simulink model "TrofazniTiristorskiIspravljac2"  (R2014b)
settings: Solver=ode5  StartTime=0.0  StopTime=0.1  FixedStep=10e-6  RelTol=1e-3
values from neighbouring files (symbols this model uses):
  alfa = 60    [ParametriSimulacije.m]
  f = 50    [ParametriSimulacije.m]
  L = 20e-3    (= 0.02)    [ParametriSimulacije.m]
  R = 10    [ParametriSimulacije.m]
  Vmax = 220*sqrt(2)    [ParametriSimulacije.m]
libraries: powerlib x13
settings Model: Creator=Zorana  LastModifiedBy=Zorana

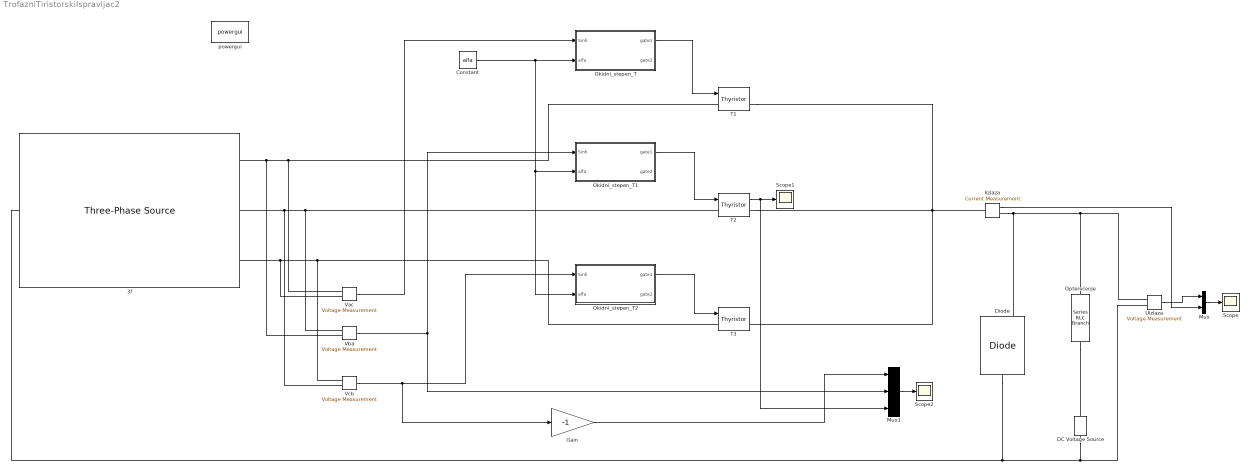
== system TrofazniTiristorskiIspravljac2 ==
  3f : powerlib/Electrical Sources/Three-Phase Source  Voltage=380  PhaseAngle=0  Frequency=f  InternalConnection=Yn  SpecifyImpedance=off  Resistance=1e-6  Inductance=0  ShortCircuitLevel=100e6  BaseVoltage=25e3  XRratio=7  BusType=swing  Pref=0  Qref=0  Qmin=-inf  Qmax=inf
  Constant : Constant  Value=alfa
  DC Voltage Source : powerlib/Electrical Sources/DC Voltage Source  Amplitude=50  Measurements=None
  Diode : powerlib/Power Electronics/Diode  Ron=1e-6  Lon=0  Vf=0  IC=0  UseSnubber=off  Rs=500  Cs=250e-9  Measurements=on
  Gain : Gain  Gain=-1
  Iizlaza : powerlib/Measurements/Current Measurement  PhasorSimulation=off  OutputType=Complex  PSBequivalent=0
  Mux : Mux  Inputs=2
  Mux1 : Mux  Inputs=3
  Okidni_stepen_T : Subsystem
  Okidni_stepen_T1 : Subsystem
  Okidni_stepen_T2 : Subsystem
  Opterećenje : powerlib/Elements/Series RLC Branch  LConnTagsString=__new0  RConnTagsString=__new0  BranchType=RL  Resistance=R  Inductance=L  SetiL0=off  InitialCurrent=0  Capacitance=1e-6  Setx0=off  InitialVoltage=0  Measurements=None
  Scope : Scope
  Scope1 : Scope
  Scope2 : Scope
      settings: SaveName=ScopeData2
  T1 : powerlib/Power Electronics/Thyristor  Ron=1e-6  Lon=0  Vf=0  IC=0  Rs=500  Cs=250e-9  Measurements=on
  T2 : powerlib/Power Electronics/Thyristor  Ron=1e-6  Lon=0  Vf=0  IC=0  Rs=500  Cs=250e-9  Measurements=on
  T3 : powerlib/Power Electronics/Thyristor  Ron=1e-6  Lon=0  Vf=0  IC=0  Rs=500  Cs=250e-9  Measurements=on
  Uizlaza : powerlib/Measurements/Voltage Measurement  PhasorSimulation=off  OutputType=Complex  PSBequivalent=0
  Vac : powerlib/Measurements/Voltage Measurement  PhasorSimulation=off  OutputType=Complex  PSBequivalent=0
  Vba : powerlib/Measurements/Voltage Measurement  PhasorSimulation=off  OutputType=Complex  PSBequivalent=0
  Vcb : powerlib/Measurements/Voltage Measurement  PhasorSimulation=off  OutputType=Complex  PSBequivalent=0
  powergui : powerlib/powergui  Priority=1  SimulationMode=Continuous  SolverType=Tustin/Backward Euler (TBE)  SampleTime=50e-6  frequency=60  SPID=off  DisableSnubberDevices=off  DisableRonSwitches=off  DisableVfSwitches=off  SwTol=0  DisplayEquations=off  Interpol=off  methode=off  Ts=100  frequencyindice=50  Pbase=100e6  ErrMax=1e-4  Iterations=50  UnitsV=kV  UnitsW=MW  FunctionMessages=off  echomessages=off  HookPort=off  EnableUseOfTLC=off  x0status=blocks  RestoreLinks=warning  ResistiveCurrentMeasurement=off  Frange=[0:2:500]  Ylog=off  Xlog=on  ShowGrid=off  save=off  variable=ZData  structure=0  ZoomFFT=off  StartTime=0.0  cycles=1  DisplayStyle=1  fundamental=60  FreqAxis=off  MaxFrequency=1000  frequencyindicesteady=1  RmsSteady=1  display=off
  wires:
  Constant/1 -> Okidni_stepen_T2/2(alfa), Okidni_stepen_T1/2(alfa), Okidni_stepen_T/2(alfa)
  Okidni_stepen_T/1(gate1) -> T1/1
  Okidni_stepen_T1/1(gate1) -> T2/1
  Okidni_stepen_T2/1(gate1) -> T3/1
  Vac/1 -> Okidni_stepen_T/1(Sinh)
  Vba/1 -> Okidni_stepen_T1/1(Sinh), Mux1/2
  Vcb/1 -> Gain/1, Okidni_stepen_T2/1(Sinh)
  Uizlaza/1 -> Mux/1
  Mux/1 -> Scope/1
  Iizlaza/1 -> Mux/2
  T2/1 -> Mux1/3, Scope1/1
  Mux1/1 -> Scope2/1
  Gain/1 -> Mux1/1
  connections:
  T1/LConn1 -- Vac/LConn1 -- Vba/LConn2 -- 3f/RConn1
  T2/LConn1 -- Vba/LConn1 -- 3f/RConn2 -- Vcb/LConn2
  T3/LConn1 -- Vcb/LConn1 -- Vac/LConn2 -- 3f/RConn3
  T1/RConn1 -- Iizlaza/LConn1 -- T2/RConn1 -- T3/RConn1
  Uizlaza/LConn2 -- DC Voltage Source/LConn1 -- Diode/LConn1 -- 3f/LConn1
  Iizlaza/RConn1 -- Uizlaza/LConn1 -- Opterećenje/LConn1 -- Diode/RConn1
  Opterećenje/RConn1 -- DC Voltage Source/RConn1

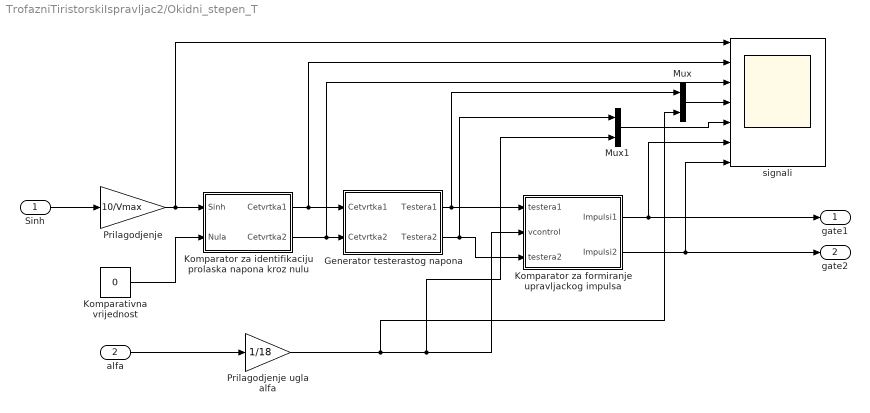
== system TrofazniTiristorskiIspravljac2/Okidni_stepen_T ==
  Sinh : Inport
  alfa : Inport  Port=2
  Generator testerastog napona : Subsystem
  Komparativna vrijednost : Constant  Value=0
  Komparator za formiranje upravljackog impulsa : Subsystem
  Komparator za identifikaciju prolaska napona kroz nulu : Subsystem
  Mux : Mux  Inputs=2
  Mux1 : Mux  Inputs=2
  Prilagodjenje : Gain  Gain=10/Vmax
  Prilagodjenje ugla alfa : Gain  Gain=1/18
  signali : Scope  NumInputPorts=7
      settings: YMin=-10~0~0~0~-5~0~0  YMax=10~11~11~11~5~11~11  SaveName=ScopeData3
  gate1 : Outport
  gate2 : Outport  Port=2
  wires:
  Komparator za formiranje upravljackog impulsa/1(Impulsi1) -> signali/6, gate1/1
  Komparator za identifikaciju prolaska napona kroz nulu/1(Cetvrtka1) -> signali/2, Generator testerastog napona/1(Cetvrtka1)
  Sinh/1 -> Prilagodjenje/1
  Prilagodjenje ugla alfa/1 -> Mux/2, Mux1/2, Komparator za formiranje upravljackog impulsa/2(vcontrol)
  Prilagodjenje/1 -> signali/1, Komparator za identifikaciju prolaska napona kroz nulu/1(Sinh)
  Generator testerastog napona/1(Testera1) -> Mux/1, Komparator za formiranje upravljackog impulsa/1(testera1)
  alfa/1 -> Prilagodjenje ugla alfa/1
  Komparativna vrijednost/1 -> Komparator za identifikaciju prolaska napona kroz nulu/2(Nula)
  Komparator za identifikaciju prolaska napona kroz nulu/2(Cetvrtka2) -> signali/3, Generator testerastog napona/2(Cetvrtka2)
  Generator testerastog napona/2(Testera2) -> Mux1/1, Komparator za formiranje upravljackog impulsa/3(testera2)
  Komparator za formiranje upravljackog impulsa/2(Impulsi2) -> signali/7, gate2/1
  Mux/1 -> signali/4
  Mux1/1 -> signali/5

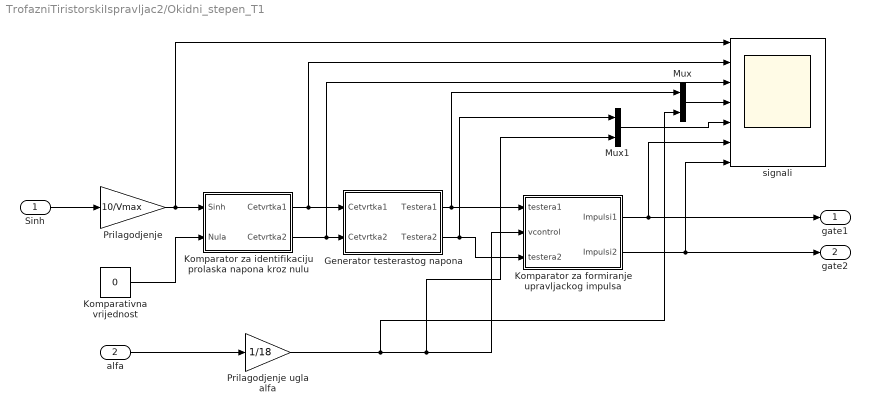
== system TrofazniTiristorskiIspravljac2/Okidni_stepen_T1 ==
  Sinh : Inport
  alfa : Inport  Port=2
  Generator testerastog napona : Subsystem
  Komparativna vrijednost : Constant  Value=0
  Komparator za formiranje upravljackog impulsa : Subsystem
  Komparator za identifikaciju prolaska napona kroz nulu : Subsystem
  Mux : Mux  Inputs=2
  Mux1 : Mux  Inputs=2
  Prilagodjenje : Gain  Gain=10/Vmax
  Prilagodjenje ugla alfa : Gain  Gain=1/18
  signali : Scope  NumInputPorts=7
      settings: YMin=-10~0~0~0~-5~0~0  YMax=10~11~11~11~5~11~11  SaveName=ScopeData3
  gate1 : Outport
  gate2 : Outport  Port=2
  wires:
  Mux1/1 -> signali/5
  Mux/1 -> signali/4
  Komparator za formiranje upravljackog impulsa/2(Impulsi2) -> gate2/1, signali/7
  Generator testerastog napona/2(Testera2) -> Komparator za formiranje upravljackog impulsa/3(testera2), Mux1/1
  Komparator za identifikaciju prolaska napona kroz nulu/2(Cetvrtka2) -> Generator testerastog napona/2(Cetvrtka2), signali/3
  Komparativna vrijednost/1 -> Komparator za identifikaciju prolaska napona kroz nulu/2(Nula)
  alfa/1 -> Prilagodjenje ugla alfa/1
  Generator testerastog napona/1(Testera1) -> Komparator za formiranje upravljackog impulsa/1(testera1), Mux/1
  Prilagodjenje/1 -> Komparator za identifikaciju prolaska napona kroz nulu/1(Sinh), signali/1
  Prilagodjenje ugla alfa/1 -> Komparator za formiranje upravljackog impulsa/2(vcontrol), Mux1/2, Mux/2
  Sinh/1 -> Prilagodjenje/1
  Komparator za identifikaciju prolaska napona kroz nulu/1(Cetvrtka1) -> Generator testerastog napona/1(Cetvrtka1), signali/2
  Komparator za formiranje upravljackog impulsa/1(Impulsi1) -> gate1/1, signali/6

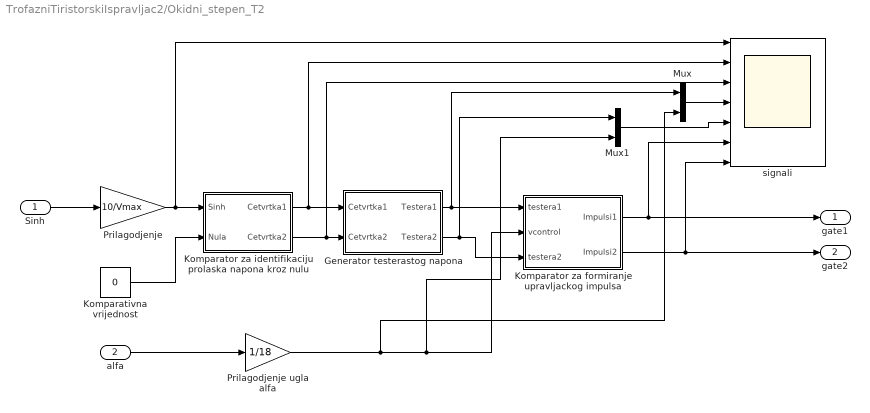
== system TrofazniTiristorskiIspravljac2/Okidni_stepen_T2 ==
  Sinh : Inport
  alfa : Inport  Port=2
  Generator testerastog napona : Subsystem
  Komparativna vrijednost : Constant  Value=0
  Komparator za formiranje upravljackog impulsa : Subsystem
  Komparator za identifikaciju prolaska napona kroz nulu : Subsystem
  Mux : Mux  Inputs=2
  Mux1 : Mux  Inputs=2
  Prilagodjenje : Gain  Gain=10/Vmax
  Prilagodjenje ugla alfa : Gain  Gain=1/18
  signali : Scope  NumInputPorts=7
      settings: YMin=-10~0~0~0~-5~0~0  YMax=10~11~11~11~5~11~11  SaveName=ScopeData3
  gate1 : Outport
  gate2 : Outport  Port=2
  wires:
  Komparator za formiranje upravljackog impulsa/1(Impulsi1) -> signali/6, gate1/1
  Komparator za identifikaciju prolaska napona kroz nulu/1(Cetvrtka1) -> signali/2, Generator testerastog napona/1(Cetvrtka1)
  Sinh/1 -> Prilagodjenje/1
  Prilagodjenje ugla alfa/1 -> Mux/2, Mux1/2, Komparator za formiranje upravljackog impulsa/2(vcontrol)
  Prilagodjenje/1 -> signali/1, Komparator za identifikaciju prolaska napona kroz nulu/1(Sinh)
  Generator testerastog napona/1(Testera1) -> Mux/1, Komparator za formiranje upravljackog impulsa/1(testera1)
  alfa/1 -> Prilagodjenje ugla alfa/1
  Komparativna vrijednost/1 -> Komparator za identifikaciju prolaska napona kroz nulu/2(Nula)
  Komparator za identifikaciju prolaska napona kroz nulu/2(Cetvrtka2) -> signali/3, Generator testerastog napona/2(Cetvrtka2)
  Generator testerastog napona/2(Testera2) -> Mux1/1, Komparator za formiranje upravljackog impulsa/3(testera2)
  Komparator za formiranje upravljackog impulsa/2(Impulsi2) -> signali/7, gate2/1
  Mux/1 -> signali/4
  Mux1/1 -> signali/5

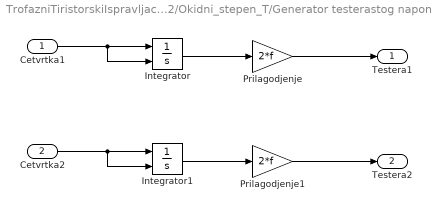
== system TrofazniTiristorskiIspravljac2/Okidni_stepen_T/Generator testerastog napona ==
  Cetvrtka1 : Inport
  Cetvrtka2 : Inport  Port=2
  Integrator : Integrator  ExternalReset=either
  Integrator1 : Integrator  ExternalReset=either
  Prilagodjenje : Gain  Gain=2*f
  Prilagodjenje1 : Gain  Gain=2*f
  Testera1 : Outport
  Testera2 : Outport  Port=2
  wires:
  Integrator/1 -> Prilagodjenje/1
  Cetvrtka1/1 -> Integrator/1, Integrator/2
  Prilagodjenje/1 -> Testera1/1
  Integrator1/1 -> Prilagodjenje1/1
  Cetvrtka2/1 -> Integrator1/2, Integrator1/1
  Prilagodjenje1/1 -> Testera2/1

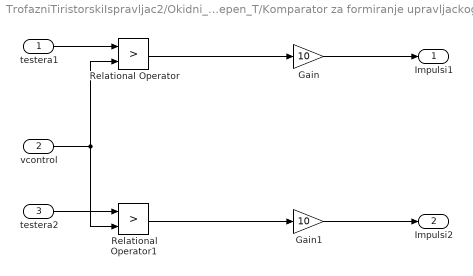
== system TrofazniTiristorskiIspravljac2/Okidni_stepen_T/Komparator za formiranje upravljackog impulsa ==
  testera1 : Inport
  vcontrol : Inport  Port=2
  testera2 : Inport  Port=3
  Gain : Gain  Gain=10
  Gain1 : Gain  Gain=10
  Relational Operator : RelationalOperator  Operator=>  OutDataTypeStr=fixdt(1,16)  InputSameDT=on
  Relational Operator1 : RelationalOperator  Operator=>  OutDataTypeStr=fixdt(1,16)  InputSameDT=on
  Impulsi1 : Outport
  Impulsi2 : Outport  Port=2
  wires:
  vcontrol/1 -> Relational Operator/2, Relational Operator1/2
  testera1/1 -> Relational Operator/1
  Gain/1 -> Impulsi1/1
  testera2/1 -> Relational Operator1/1
  Gain1/1 -> Impulsi2/1
  Relational Operator/1 -> Gain/1
  Relational Operator1/1 -> Gain1/1

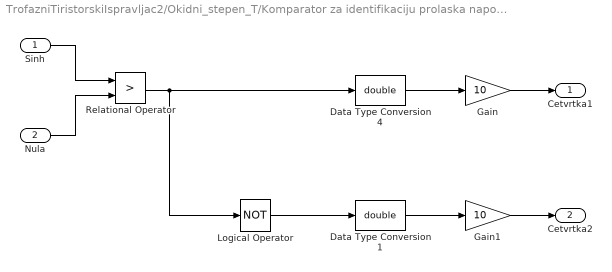
== system TrofazniTiristorskiIspravljac2/Okidni_stepen_T/Komparator za identifikaciju prolaska napona kroz nulu ==
  Sinh : Inport
  Nula : Inport  Port=2
  Data Type Conversion1 : DataTypeConversion  OutDataTypeStr=double  SaturateOnIntegerOverflow=on  RndMeth=Zero
  Data Type Conversion4 : DataTypeConversion  OutDataTypeStr=double  SaturateOnIntegerOverflow=on  RndMeth=Zero
  Gain : Gain  Gain=10
  Gain1 : Gain  Gain=10
  Logical Operator : Logic  Operator=NOT  IconShape=distinctive  AllPortsSameDT=off  OutDataTypeStr=boolean
  Relational Operator : RelationalOperator  Operator=>  OutDataTypeStr=fixdt(1,16)  InputSameDT=on
  Cetvrtka1 : Outport
  Cetvrtka2 : Outport  Port=2
  wires:
  Gain/1 -> Cetvrtka1/1
  Sinh/1 -> Relational Operator/1
  Nula/1 -> Relational Operator/2
  Relational Operator/1 -> Logical Operator/1, Data Type Conversion4/1
  Data Type Conversion4/1 -> Gain/1
  Gain1/1 -> Cetvrtka2/1
  Data Type Conversion1/1 -> Gain1/1
  Logical Operator/1 -> Data Type Conversion1/1

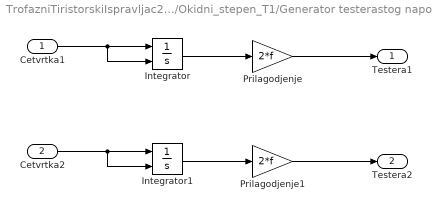
== system TrofazniTiristorskiIspravljac2/Okidni_stepen_T1/Generator testerastog napona ==
  Cetvrtka1 : Inport
  Cetvrtka2 : Inport  Port=2
  Integrator : Integrator  ExternalReset=either
  Integrator1 : Integrator  ExternalReset=either
  Prilagodjenje : Gain  Gain=2*f
  Prilagodjenje1 : Gain  Gain=2*f
  Testera1 : Outport
  Testera2 : Outport  Port=2
  wires:
  Prilagodjenje1/1 -> Testera2/1
  Cetvrtka2/1 -> Integrator1/1, Integrator1/2
  Integrator1/1 -> Prilagodjenje1/1
  Prilagodjenje/1 -> Testera1/1
  Cetvrtka1/1 -> Integrator/2, Integrator/1
  Integrator/1 -> Prilagodjenje/1

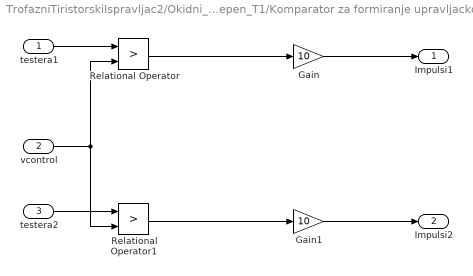
== system TrofazniTiristorskiIspravljac2/Okidni_stepen_T1/Komparator za formiranje upravljackog impulsa ==
  testera1 : Inport
  vcontrol : Inport  Port=2
  testera2 : Inport  Port=3
  Gain : Gain  Gain=10
  Gain1 : Gain  Gain=10
  Relational Operator : RelationalOperator  Operator=>  OutDataTypeStr=fixdt(1,16)  InputSameDT=on
  Relational Operator1 : RelationalOperator  Operator=>  OutDataTypeStr=fixdt(1,16)  InputSameDT=on
  Impulsi1 : Outport
  Impulsi2 : Outport  Port=2
  wires:
  Relational Operator1/1 -> Gain1/1
  Relational Operator/1 -> Gain/1
  Gain1/1 -> Impulsi2/1
  testera2/1 -> Relational Operator1/1
  Gain/1 -> Impulsi1/1
  testera1/1 -> Relational Operator/1
  vcontrol/1 -> Relational Operator1/2, Relational Operator/2

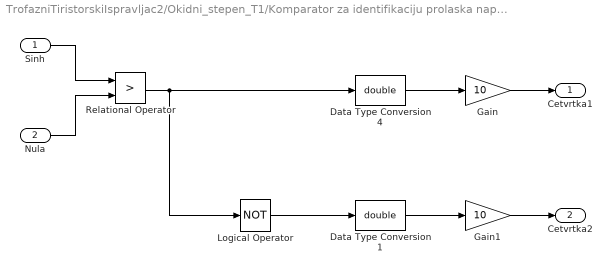
== system TrofazniTiristorskiIspravljac2/Okidni_stepen_T1/Komparator za identifikaciju prolaska napona kroz nulu ==
  Sinh : Inport
  Nula : Inport  Port=2
  Data Type Conversion1 : DataTypeConversion  OutDataTypeStr=double  SaturateOnIntegerOverflow=on  RndMeth=Zero
  Data Type Conversion4 : DataTypeConversion  OutDataTypeStr=double  SaturateOnIntegerOverflow=on  RndMeth=Zero
  Gain : Gain  Gain=10
  Gain1 : Gain  Gain=10
  Logical Operator : Logic  Operator=NOT  IconShape=distinctive  AllPortsSameDT=off  OutDataTypeStr=boolean
  Relational Operator : RelationalOperator  Operator=>  OutDataTypeStr=fixdt(1,16)  InputSameDT=on
  Cetvrtka1 : Outport
  Cetvrtka2 : Outport  Port=2
  wires:
  Logical Operator/1 -> Data Type Conversion1/1
  Data Type Conversion1/1 -> Gain1/1
  Gain1/1 -> Cetvrtka2/1
  Data Type Conversion4/1 -> Gain/1
  Relational Operator/1 -> Data Type Conversion4/1, Logical Operator/1
  Nula/1 -> Relational Operator/2
  Sinh/1 -> Relational Operator/1
  Gain/1 -> Cetvrtka1/1

== system TrofazniTiristorskiIspravljac2/Okidni_stepen_T2/Generator testerastog napona ==
  Cetvrtka1 : Inport
  Cetvrtka2 : Inport  Port=2
  Integrator : Integrator  ExternalReset=either
  Integrator1 : Integrator  ExternalReset=either
  Prilagodjenje : Gain  Gain=2*f
  Prilagodjenje1 : Gain  Gain=2*f
  Testera1 : Outport
  Testera2 : Outport  Port=2
  wires:
  Integrator/1 -> Prilagodjenje/1
  Cetvrtka1/1 -> Integrator/1, Integrator/2
  Prilagodjenje/1 -> Testera1/1
  Integrator1/1 -> Prilagodjenje1/1
  Cetvrtka2/1 -> Integrator1/2, Integrator1/1
  Prilagodjenje1/1 -> Testera2/1

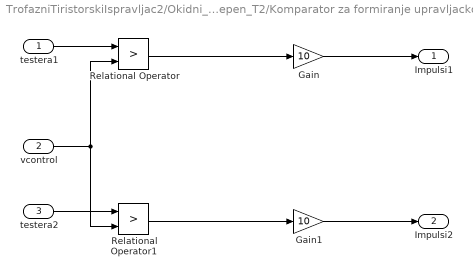
== system TrofazniTiristorskiIspravljac2/Okidni_stepen_T2/Komparator za formiranje upravljackog impulsa ==
  testera1 : Inport
  vcontrol : Inport  Port=2
  testera2 : Inport  Port=3
  Gain : Gain  Gain=10
  Gain1 : Gain  Gain=10
  Relational Operator : RelationalOperator  Operator=>  OutDataTypeStr=fixdt(1,16)  InputSameDT=on
  Relational Operator1 : RelationalOperator  Operator=>  OutDataTypeStr=fixdt(1,16)  InputSameDT=on
  Impulsi1 : Outport
  Impulsi2 : Outport  Port=2
  wires:
  vcontrol/1 -> Relational Operator/2, Relational Operator1/2
  testera1/1 -> Relational Operator/1
  Gain/1 -> Impulsi1/1
  testera2/1 -> Relational Operator1/1
  Gain1/1 -> Impulsi2/1
  Relational Operator/1 -> Gain/1
  Relational Operator1/1 -> Gain1/1

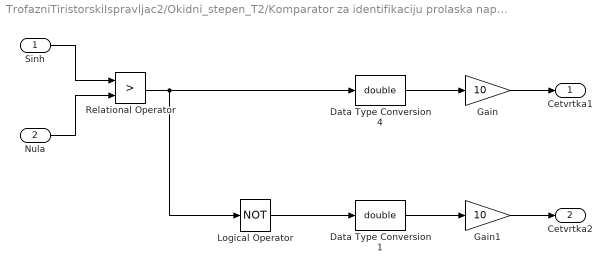
== system TrofazniTiristorskiIspravljac2/Okidni_stepen_T2/Komparator za identifikaciju prolaska napona kroz nulu ==
  Sinh : Inport
  Nula : Inport  Port=2
  Data Type Conversion1 : DataTypeConversion  OutDataTypeStr=double  SaturateOnIntegerOverflow=on  RndMeth=Zero
  Data Type Conversion4 : DataTypeConversion  OutDataTypeStr=double  SaturateOnIntegerOverflow=on  RndMeth=Zero
  Gain : Gain  Gain=10
  Gain1 : Gain  Gain=10
  Logical Operator : Logic  Operator=NOT  IconShape=distinctive  AllPortsSameDT=off  OutDataTypeStr=boolean
  Relational Operator : RelationalOperator  Operator=>  OutDataTypeStr=fixdt(1,16)  InputSameDT=on
  Cetvrtka1 : Outport
  Cetvrtka2 : Outport  Port=2
  wires:
  Gain/1 -> Cetvrtka1/1
  Sinh/1 -> Relational Operator/1
  Nula/1 -> Relational Operator/2
  Relational Operator/1 -> Logical Operator/1, Data Type Conversion4/1
  Data Type Conversion4/1 -> Gain/1
  Gain1/1 -> Cetvrtka2/1
  Data Type Conversion1/1 -> Gain1/1
  Logical Operator/1 -> Data Type Conversion1/1
